simulink model "SYT_A28_mod"  (Simulink 7.0)
settings: Solver=ode4  StartTime=0.0  StopTime=40.0  FixedStep=0.1  RelTol=1e-3
values from neighbouring files (symbols this model uses):
  T = 2    [a06.m]    (also in a22.m = 10; a27.m = 1; a28.m = 0.1; a29.m = 0.1)
settings Model: Creator=Volker  LastModifiedBy=Volker
settings DataIOCC: SignalLoggingName=sigsOut
settings DebuggingCC: SaveWithParameterizedLinksMsg=none  SignalResolutionControl=TryResolveAllWithWarning  SolverPrmCheckMsg=none  MultiTaskDSMMsg=warning  MultiTaskCondExecSysMsg=none  StrictBusMsg=None
settings HardwareCC: TargetUnknown=on
settings RTWCC: IncludeERTFirstTime=on

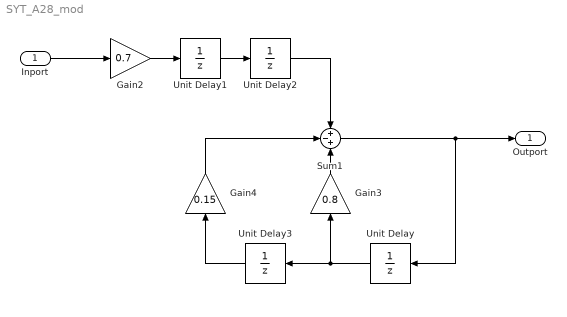
== system SYT_A28_mod ==
  Inport : Inport  OutDataType=sfix(16)  OutScaling=2^0
  Gain2 : Gain  Gain=0.7  ParameterDataType=sfix(16)  ParameterScaling=2^0  OutDataType=sfix(16)  OutScaling=2^0  SaturateOnIntegerOverflow=on
  Gain3 : Gain  Orientation=up  Gain=0.8  ParameterDataType=sfix(16)  ParameterScaling=2^0  OutDataType=sfix(16)  OutScaling=2^0  SaturateOnIntegerOverflow=on
  Gain4 : Gain  Orientation=up  Gain=0.15  ParameterDataType=sfix(16)  ParameterScaling=2^0  OutDataType=sfix(16)  OutScaling=2^0  SaturateOnIntegerOverflow=on
  Sum1 : Sum  Inputs=+-+  OutDataType=sfix(16)  OutScaling=2^0  SaturateOnIntegerOverflow=on  InputSameDT=on
  Unit Delay : UnitDelay  Orientation=left  SampleTime=T
  Unit Delay1 : UnitDelay  SampleTime=T
  Unit Delay2 : UnitDelay  SampleTime=T
  Unit Delay3 : UnitDelay  Orientation=left  SampleTime=T
  Outport : Outport
  wires:
  Unit Delay1/1 -> Unit Delay2/1
  Gain2/1 -> Unit Delay1/1
  Unit Delay2/1 -> Sum1/1
  Sum1/1 -> Unit Delay/1, Outport/1
  Unit Delay/1 -> Unit Delay3/1, Gain3/1
  Gain3/1 -> Sum1/3
  Unit Delay3/1 -> Gain4/1
  Gain4/1 -> Sum1/2
  Inport/1 -> Gain2/1
